simulink model "untitled"  (R2019a)
settings: Solver=FixedStepAuto  StartTime=0.0  StopTime=inf  RelTol=1e-3
libraries: dspnetwork x1
settings Model: Creator=10291  LastModifiedBy=10291

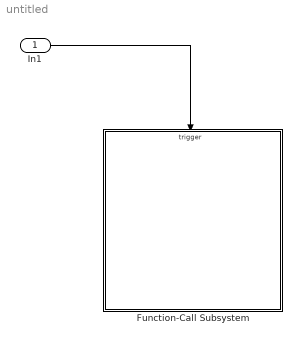
== system untitled ==
  In1 : Inport  SampleTime=0.1  OutputFunctionCall=on
  Function-Call Subsystem : Subsystem  TreatAsAtomicUnit=on
  wires:
  In1/1 -> Function-Call Subsystem/Trigger

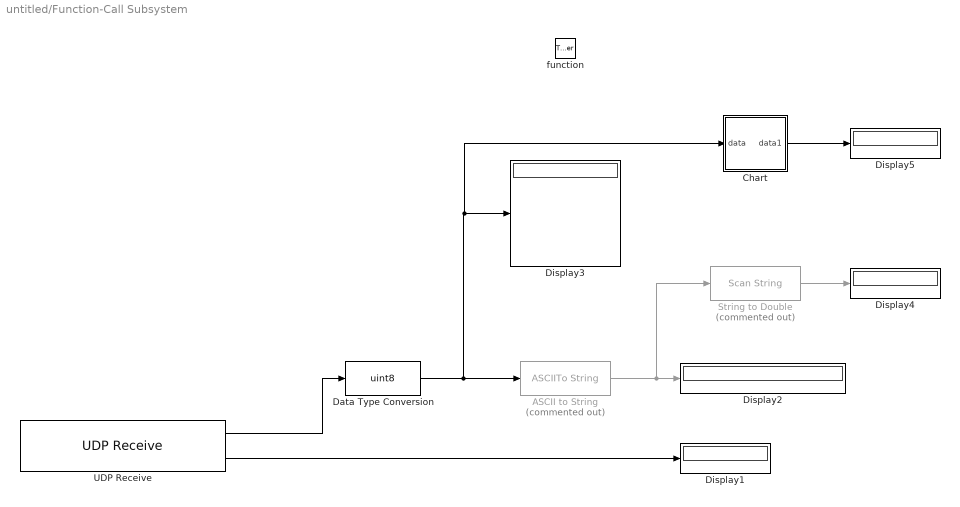
== system untitled/Function-Call Subsystem ==
  function : TriggerPort  TriggerType=function-call  VariantControl=Variant
  ASCII to String : ASCIIToString  Commented=on
  Chart : Stateflow chart  BlockKeywords=__PRM__SERIALIZED__DATA__:Stateflow Chart,Stateflow Diagram  TreatAsAtomicUnit=on
  Data Type Conversion : DataTypeConversion  OutDataTypeStr=uint8
  Display{1..5} (5 alike) : Display
      Display3 settings: Format=hex (Stored Integer)
  String to Double : ScanString  Commented=on  Format="\"%lf\""
  UDP Receive : dspnetwork/UDP Receive  localURL='0.0.0.0'  localPort=25000  remoteURL='192.168.31.126'  remotePort=-1  recvBufferSize=8192  dims=10  signalDatatype=uint8  isComplex=off  isVarSize=off  showBlockingTime=off  blockingTime=0  sampletime=-1  blockPlatform=[]
      settings: SourceProductName=Simulink
  wires:
  String to Double/1 -> Display4/1
  ASCII to String/1 -> String to Double/1, Display2/1
  UDP Receive/2 -> Display1/1
  UDP Receive/1 -> Data Type Conversion/1
  Chart/1(data1) -> Display5/1
  Data Type Conversion/1 -> Chart/1(data), Display3/1, ASCII to String/1

== stateflow chart untitled/Function-Call Subsystem/Chart ==
  (default) -> (junction 3) : {dd = ascii2str(data);}
  (junction 3) -> (junction 5) : %[data == 1]
  (junction 5) -> (junction 7) : {data1 = 1;}
  (junction 7) -> (junction 9)
  (junction 9) -> (junction 12)
  data: data input; data1 output; dd local string
